simulink model "convolution_2D_v3_int"  (R2024b)
settings: Solver=FixedStepDiscrete  StartTime=0.0  StopTime=15  RelTol=1e-3
InitFcn:
  | % Define a random matrix size between 3 and 10
  | n =4;
  | K=zeros(3);
  | for i=1:3
  |     for j=1:3
  |         K(i,j)=randi([0,100]);
  |     end
  | end
  | fprintf('Size of matrix A: n = %d\n', n);
libraries: simulink x1, hdlsllib x1
settings Model: DataTypeOverride=Off  Creator=valen  LastModifiedBy=valen
settings SolverCC: AlgebraicLoopSolver=TrustRegion  AutoInsertRateTranBlk=on
settings DataIOCC: LimitDataPoints=on  SaveOutput=off  SaveTime=off
settings OptimizationCC: BlockReduction=off  ConditionallyExecuteInputs=off  DefaultParameterBehavior=Inlined  LifeSpan=inf
settings DebuggingCC: AlgebraicLoopMsg=error  SingleTaskRateTransMsg=error  UnconnectedInputMsg=warning  UnconnectedOutputMsg=warning  UnconnectedLineMsg=warning  AllowSymbolicDim=off  StrictBusMsg=ErrorOnBusTreatedAsVector  SFUnexpectedBacktrackingDiag=warning  SFNoUnconditionalDefaultTransitionDiag=warning  SFExecutionAtInitializationDiag=none  ArithmeticOperatorsInVariantConditions=warning
settings HardwareCC: ProdBitPerPointer=32  ProdBitPerSizeT=32  ProdBitPerPtrDiffT=32  ProdLargestAtomicFloat=None  ProdIntDivRoundTo=Undefined  ProdEndianess=Unspecified  ProdWordSize=32  ProdHWDeviceType=ASIC/FPGA->ASIC/FPGA  ProdEqTarget=off
settings ModelReferenceCC: EnableRefExpFcnMdlSchedulingChecks=on
settings SFSimCC: SimUseLocalCustomCode=off  CustomCodeUndefinedFunction=UseInterfaceOnly
settings RTWCC: RTWUseLocalCustomCode=off  GPUComputeCapability=3.5
settings CodeAppCC: StateflowObjectComments=on
settings GRTTargetCC: TargetLangStandard=C89/C90 (ANSI)
settings ConfigComp: CovScope=ReferencedModels  CovMetricSettings=dw  CovSaveCumulativeToWorkspaceVar=on  CovSaveSingleToWorkspaceVar=on  CovExternalEMLEnable=off  CovSFcnEnable=off

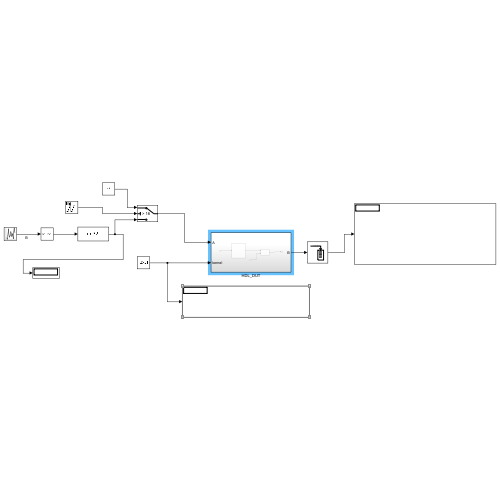
[thumbnail: Simulink's stored preview of the top-level diagram]
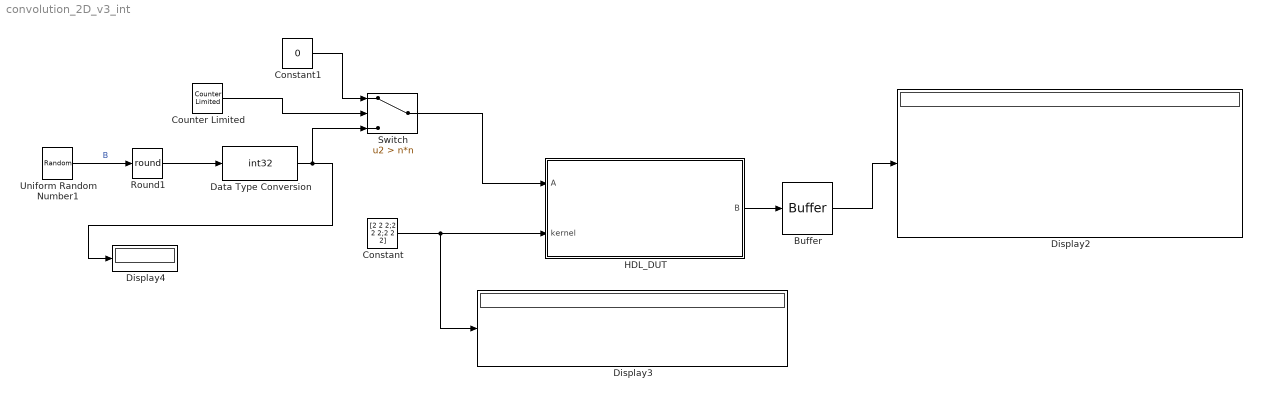
== system convolution_2D_v3_int ==
  Buffer : Buffer  N=n*n+n+1  OutputFrames=off
  Constant : Constant  Value=[2 2 2;2 2 2;2 2 2]  OutDataTypeStr=int32
  Constant1 : Constant  Value=0  OutDataTypeStr=int32
  Counter Limited : simulink/Sources/Counter Limited  uplimit=n*(n+1)  tsamp=-1
  Data Type Conversion : DataTypeConversion  OutDataTypeStr=int32  SaturateOnIntegerOverflow=off  RndMeth=Floor
  Display2 : Display
  Display3 : Display
  Display4 : Display
  HDL_DUT : Subsystem
  Round1 : Rounding  Operator=round
  Switch : Switch  Criteria=u2 > Threshold  Threshold=n*n  SaturateOnIntegerOverflow=off  InputSameDT=off
  Uniform Random Number1 : UniformRandomNumber  Minimum=0  Maximum=100  Seed=n  SampleTime=10/(n*n+1)
  wires:
  Round1/1 -> Data Type Conversion/1
  Uniform Random Number1/1 -> Round1/1  "B"
  HDL_DUT/1(B) -> Buffer/1
  Buffer/1 -> Display2/1
  Constant/1 -> Display3/1, HDL_DUT/2(kernel)
  Counter Limited/1 -> Switch/2
  Switch/1 -> HDL_DUT/1(A)
  Constant1/1 -> Switch/1
  Data Type Conversion/1 -> Display4/1, Switch/3

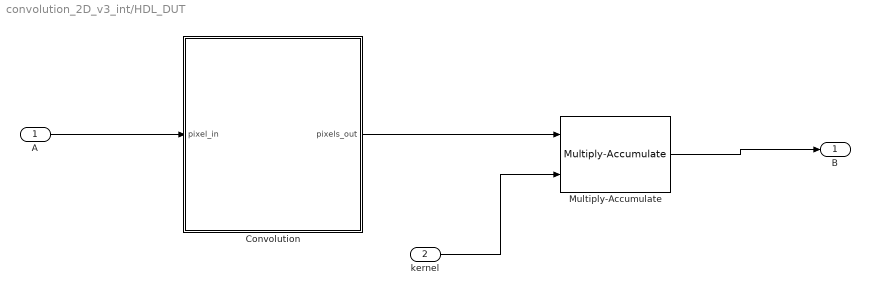
== system convolution_2D_v3_int/HDL_DUT ==
  A : Inport
  kernel : Inport  Port=2
  Convolution : MATLAB Function  TreatAsAtomicUnit=on
  Multiply-Accumulate : hdlsllib/HDL Operations/Multiply-Accumulate  opMode=Vector  initValueSetting=Dialog  initValue=0  initValueSetting2=Dialog  initValue2=0  initValueSetting3=Dialog  initValue3=0  num_samples=2  RndMeth2=Floor  RndMeth3=Floor  datatype2=Inherit: Inherit via back propagation  datatype3=Inherit: Inherit via back propagation  validOut=on  endInandOut=on  startOut=on  countOut=on  dim=-1  DoSatur=off  parallel=off
  B : Outport  VectorParamsAs1DForOutWhenUnconnected=off
  wires:
  A/1 -> Convolution/1(pixel_in)
  kernel/1 -> Multiply-Accumulate/2
  Convolution/1(pixels_out) -> Multiply-Accumulate/1
  Multiply-Accumulate/1 -> B/1

== matlab function convolution_2D_v3_int/HDL_DUT/Convolution ==
  data: pixel_in input; pixels_out output
function pixels_out = fcn(pixel_in)
    persistent line1 line2 window count;
    
    WIDTH = 4;
    TOTAL_PIXELS = WIDTH * WIDTH;
    
    % LATENCE : Nombre de cycles requis pour que le premier pixel de l'image (1,1)
    % se retrouve exactement au centre (coordonnées 2,2) de notre fenêtre 3x3.
    % Formule standard en streaming : WIDTH + 1 + 1 = WIDTH + 2
    LATENCY = WIDTH + 2; 
    
    if isempty(line1)
        line1 = zeros(1, WIDTH, 'int32'); 
        line2 = zeros(1, WIDTH, 'int32');
        window = zeros(3, 3, 'int32');
        count = int32(0); 
    end
    
    % 1. Mise à jour des registres à décalage (Streaming)
    p_l1 = line1(1); 
    p_l2 = line2(1);
    
    line1(1:WIDTH-1) = line1(2:WIDTH);
    line1(WIDTH) = int32(pixel_in);
    
    line2(1:WIDTH-1) = line2(2:WIDTH);
    line2(WIDTH) = p_l1;
    
    window(:, 1:2) = window(:, 2:3);
    window(1, 3) = p_l2;
    window(2, 3) = p_l1;
    window(3, 3) = int32(pixel_in);
    
    % Incrémentation du compteur global de pixels reçus
    count = count + 1;
    
    % 2. Détermination de la position du pixel virtuel au centre de la fenêtre
    out_count = count - LATENCY + 1;
    
    % Si on est dans la plage valide de l'image (1 à 16)
    if out_count >= 1 && out_count <= TOTAL_PIXELS
        
        % Extraction des coordonnées X (1 à 4) et Y (1 à 4) du pixel central
        out_y = floor(single(out_count - 1) / WIDTH) + 1;
        out_x = mod(single(out_count - 1), WIDTH) + 1;
        
        % On prépare la sortie avec le contenu actuel de la fenêtre
        current_window = window;
        
        % --- GESTION DES EFFETS DE BORD (ZERO PADDING) ---
        
        % Bord GAUCHE : Si le centre est sur la col 1, la col gauche du filtre (1) déborde
        if out_x == 1
            current_window(:, 1) = int32([0; 0; 0]);
        end
        
        % Bord DROIT : Si le centre est sur la col WIDTH, la col droite du filtre (3) déborde
        if out_x == WIDTH
            current_window(:, 3) = int32([0; 0; 0]);
        end
        
        % Bord HAUT : Si le centre est sur la ligne 1, la ligne du haut du filtre (1) déborde
        if out_y == 1
            current_window(1, :) = int32([0, 0, 0]);
        end
        
        % Bord BAS : Si le centre est sur la ligne WIDTH, la ligne du bas du filtre (3) déborde
        if out_y == WIDTH
            current_window(3, :) = int32([0, 0, 0]);
        end
        
        pixels_out = current_window;
    else
        % Hors de l'image (Période transitoire / Latence initiale ou finale)
        pixels_out = zeros(3, 3, 'int32');
    end
end
